simulink model "fig10_68"  (Simulink 7.0)
settings: Solver=ode45  SolverMode=SingleTasking  StartTime=0.0  StopTime=100.0  RelTol=1e-5  AbsTol=1e-6
values from neighbouring files (symbols this model uses):
  a = [f, 0*f ... (first row only)    [fig10_18.m]    (also in fig10_19.m; fig10_20.m; fig10_21.m; fig10_22.m)
  b = [g;0*g]    [fig10_18.m]    (also in fig10_19.m; fig10_20.m; fig10_21.m; fig10_22.m)
  d = [0]    [fig10_18.m]    (also in fig10_19.m; fig10_20.m; fig10_21.m; fig10_22.m)
undefined symbols (not defined in the file or in its folder): c_center
libraries: simulink x1
CloseFcn:
  | ;slview('closediagram',bdroot);
settings Model: Creator=abbas  LastModifiedBy=abbas
settings DataIOCC: LimitDataPoints=off
settings OptimizationCC: BlockReduction=off  BooleanDataType=off  InlineInvariantSignals=on
settings DebuggingCC: SaveWithParameterizedLinksMsg=none  SignalResolutionControl=TryResolveAllWithWarning  SolverPrmCheckMsg=none  MultiTaskDSMMsg=warning  MultiTaskCondExecSysMsg=none  StrictBusMsg=None
settings HardwareCC: TargetUnknown=on
settings RTWCC: IncludeERTFirstTime=on
settings GRTTargetCC: TargetFcnLib=ansi_tfl_tmw.mat  ModelReferenceCompliant=off  CompOptLevelCompliant=off  MatFileLogging=off

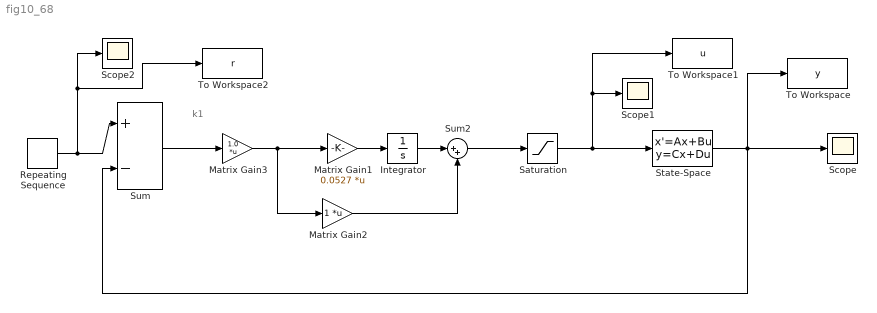
== system fig10_68 ==
  note: k1
  Integrator : Integrator
  Matrix Gain1 : Gain  Gain=0.0527  Multiplication=Matrix(K*u)  ParameterDataType=sfix(16)  ParameterScaling=2^0  OutDataType=sfix(16)  OutScaling=2^0  SaturateOnIntegerOverflow=on
  Matrix Gain2 : Gain  Multiplication=Matrix(K*u)  ParameterDataType=sfix(16)  ParameterScaling=2^0  OutDataType=sfix(16)  OutScaling=2^0  SaturateOnIntegerOverflow=on
  Matrix Gain3 : Gain  Gain=1.0  Multiplication=Matrix(K*u)  ParameterDataType=sfix(16)  ParameterScaling=2^0  OutDataType=sfix(16)  OutScaling=2^0  SaturateOnIntegerOverflow=on
  Repeating Sequence : simulink/Sources/Repeating Sequence  SystemSampleTime=-1  rep_seq_t=[0:0.1:100]  rep_seq_y=[0:.1:25 25*ones(1,500) 0*ones(1,250)]
  Saturation : Saturate  UpperLimit=100  LowerLimit=-100
  Scope : Scope
      settings: TickLabels=on  TimeRange=100  YMin=0  YMax=100  DataFormat=Array
  Scope1 : Scope
      settings: TickLabels=on  DataFormat=Array
  Scope2 : Scope
      settings: TickLabels=on  DataFormat=Array
  State-Space : StateSpace  A=a  B=b  C=c_center  D=d
  Sum : Sum  Inputs=+-  OutDataType=sfix(16)  OutScaling=2^0  SaturateOnIntegerOverflow=on  InputSameDT=on
  Sum2 : Sum  Inputs=|++  OutDataType=sfix(16)  OutScaling=2^0  SaturateOnIntegerOverflow=on  InputSameDT=on
  To Workspace : ToWorkspace  VariableName=y  SampleTime=-1  SaveFormat=Array
  To Workspace1 : ToWorkspace  VariableName=u  SampleTime=-1  SaveFormat=Array
  To Workspace2 : ToWorkspace  VariableName=r  SampleTime=-1  SaveFormat=Array
  wires:
  Matrix Gain1/1 -> Integrator/1
  State-Space/1 -> Scope/1, Sum/2, To Workspace/1
  Matrix Gain2/1 -> Sum2/2
  Integrator/1 -> Sum2/1
  Sum2/1 -> Saturation/1
  Saturation/1 -> State-Space/1, Scope1/1, To Workspace1/1
  Sum/1 -> Matrix Gain3/1
  Matrix Gain3/1 -> Matrix Gain1/1, Matrix Gain2/1
  Repeating Sequence/1 -> Sum/1, Scope2/1, To Workspace2/1
